simulink model "MCR2_Example_Publisher"  (R2024a)
settings: Solver=VariableStepAuto  StartTime=0.0  StopTime=Inf  RelTol=1e-3
libraries: robotlib x2
settings Model: Creator=mario  LastModifiedBy=mario

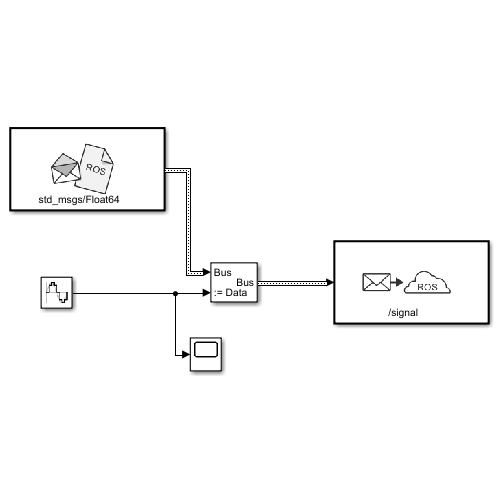
[thumbnail: Simulink's stored preview of the top-level diagram]
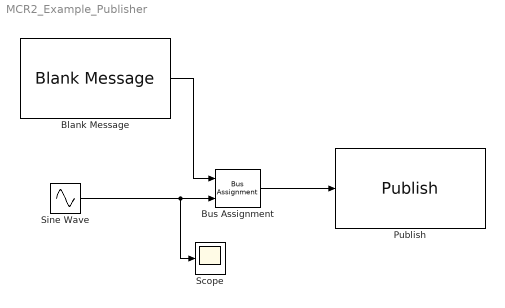
== system MCR2_Example_Publisher ==
  Blank Message : robotlib/Blank Message  messageClass=Message  entityType=std_msgs/Float64  messageType=std_msgs/Float64  SampleTime=0.01  legacyBusStruct=off
  Bus Assignment : BusAssignment  AssignedSignals=Data
  Publish : robotlib/Publish  topicSource=Specify your own  topic=/signal  messageType=std_msgs/Float64  legacyBusStruct=off  messageQueueLength=1
  Scope : Scope
  Sine Wave : Sin  SampleTime=0.01
  wires:
  Sine Wave/1 -> Scope/1, Bus Assignment/2
  Bus Assignment/1 -> Publish/1
  Blank Message/1 -> Bus Assignment/1
